simulink model "proportional_valve"  (R2023a)
settings: Solver=VariableStepAuto  StartTime=0.0  StopTime=20  RelTol=1e-3
values from neighbouring files (symbols this model uses):
  K_0V = leakage_flow / sqrt(closed_pressure_difference)    [system_parameters.m]
  K_10V = 40 / (60000 * sqrt(35e5))    [system_parameters.m]
libraries: simulink x1
settings Model: Creator=porterf1  LastModifiedBy=porterf1

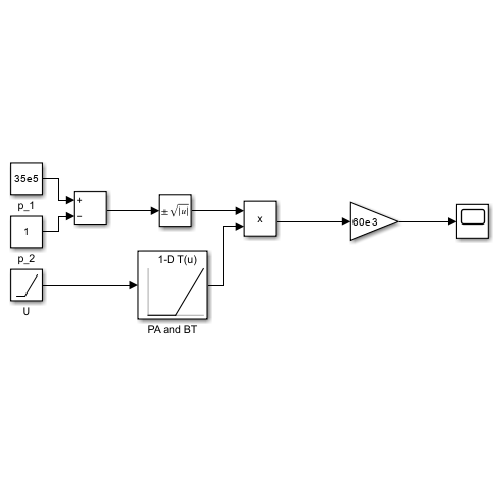
[thumbnail: Simulink's stored preview of the top-level diagram]
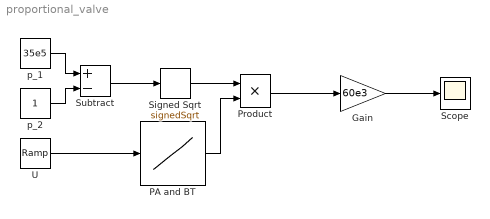
== system proportional_valve ==
  Gain : Gain  Gain=60e3
  PA and BT : Lookup_n-D  NumberOfTableDimensions=1  BreakpointsForDimension1=[-10, 0, 10]  Table=[0, K_0V, K_10V]  InternalRulePriority=Speed  RndMeth=Simplest
  Product : Product
  Scope : Scope
  Signed Sqrt : Sqrt  Operator=signedSqrt
  Subtract : Sum  Inputs=+-
  U : simulink/Sources/Ramp  slope=1  start=0  InitialOutput=-10
  p_1 : Constant  Value=35e5
  p_2 : Constant
  wires:
  p_1/1 -> Subtract/1
  p_2/1 -> Subtract/2
  Product/1 -> Gain/1
  U/1 -> PA and BT/1
  PA and BT/1 -> Product/2
  Subtract/1 -> Signed Sqrt/1
  Signed Sqrt/1 -> Product/1
  Gain/1 -> Scope/1
